simulink library "AEMS_Standard_Library"  (R2016b)
settings: Solver=ode45  StartTime=0.0  StopTime=10.0  RelTol=1e-3
undefined symbols (not defined in the file or in its folder): BkPY, carto, Cbx_extegr, Cbx_lpegrsys, Cbx_portegr, Cnx_bnk_nr_conf, Cnx_cyl_nr_conf, ConfigManagement, configuration_management, Cxx_dcm_io_tmr_end_xxxx, Cxx_dcm_rt_tmr_end, Cxx_DID_xxxx_IO_max, Cxx_DID_xxxx_IO_min, Cxx_egrhsofs, Cxx_vmaniegi, DEM_DEBOUNCE_FREEZE, DEM_DTR_CTL_INVISIBLE, DEM_DTR_CTL_NORMAL, Dem_DtrId2_XXX, Dem_DtrId3_XXX, Dem_DtrId4_XXX, Dem_DtrId5_XXX, Dem_DtrId6_XXX, Dem_DtrId7_XXX, Dem_DtrId8_XXX, Dem_DtrId9_XXX, Dem_DtrId_XXX, Dem_EnableConditionId2_XXX, Dem_EnableConditionId3_XXX, Dem_EnableConditionId4_XXX, Dem_EnableConditionId5_XXX, Dem_EnableConditionId6_XXX, Dem_EnableConditionId7_XXX, Dem_EnableConditionId8_XXX, Dem_EnableConditionId_XXX, Dem_EventId, Dem_EventId2_XXX, Dem_EventId3_XXX, Dem_EventId4_XXX, Dem_EventId5_XXX, Dem_EventId6_XXX, Dem_EventId7_XXX, Dem_EventId8_XXX, Dem_EventId9_XXX, Dem_EventId_Device_Faulttype, Dem_EventId_XXX, DEM_IUMPR_GENERAL_DENOMINATOR, DEM_OPCYC_IGNITION, Dem_RatioId2_XXX, Dem_RatioId3_XXX, Dem_RatioId4_XXX, Dem_RatioId5_XXX, Dem_RatioId6_XXX, Dem_RatioId7_XXX, Dem_RatioId8_XXX, Dem_RatioId_XXX, Dem_StorageConditionId2_XXX, Dem_StorageConditionId3_XXX, Dem_StorageConditionId4_XXX, Dem_StorageConditionId5_XXX ... (+65)
libraries: AEMS_Standard_Library x477, simulink x2
(part 38 of 39)

== system AEMS_Standard_Library/SPECIFIC/AEMS_AT_EHR/A_Enabled_Calculation/B_Temp_calculation_in_brick/C_Temp_and_power_calculation ==
  Vxx_ehr_exo_temp_flu : Inport
  Vxx_ehr_wht_temp_flu : Inport  Port=2
  Vxx_ehr_ex_gas_temp_flu : Inport  Port=3
  Vxx_ehr_ext_cnvt_temp_flu : Inport  Port=4
  Vxx_ehr_sel_tenv : Inport  Port=5
  Vxx_ehr_samp_t : Inport  Port=6
  Vxx_ehr_ext_cnvt_entr : Inport  Port=7
  Constant1 : Constant  Value=0  OutDataTypeStr=Inherit: Inherit via back propagation
  DivisionByZero : Subsystem
  Product2 : Product  OutDataTypeStr=Inherit: Inherit via back propagation  RndMeth=Zero
  Saturation : Saturate  UpperLimit=1473  LowerLimit=233  RndMeth=Zero
      settings: AttributesFormatString=<limits=%<UpperLimit>/%<LowerLimit>>
  Sum : Sum  Inputs=+-  OutDataTypeStr=Inherit: Inherit via back propagation  RndMeth=Zero  InputSameDT=on
  Sum1 : Sum  Inputs=2  OutDataTypeStr=Inherit: Inherit via back propagation  RndMeth=Zero  InputSameDT=on
  Sum2 : Sum  Inputs=2  OutDataTypeStr=Inherit: Inherit via back propagation  RndMeth=Zero  InputSameDT=on
  Sum3 : Sum  Inputs=2  OutDataTypeStr=Inherit: Inherit via back propagation  RndMeth=Zero  InputSameDT=on
  Vxx_ehr_ext_pow_loss : Outport
  Vxx_ehr_dtp : Outport  Port=2
  wires:
  Saturation/1 -> Vxx_ehr_dtp/1, Sum/1
  Sum3/1 -> Saturation/1
  Sum2/1 -> Sum3/2
  Sum1/1 -> Sum3/1
  Vxx_ehr_ext_cnvt_entr/1 -> DivisionByZero/2(Vxx_ehr_ext_cnvt_entr)
  Vxx_ehr_samp_t/1 -> DivisionByZero/1(Vxx_ehr_samp_t)
  Vxx_ehr_sel_tenv/1 -> Sum/2
  Sum/1 -> Product2/1
  DivisionByZero/1(ans) -> Product2/2
  Product2/1 -> Vxx_ehr_ext_pow_loss/1
  Vxx_ehr_exo_temp_flu/1 -> Sum1/1
  Vxx_ehr_wht_temp_flu/1 -> Sum1/2
  Vxx_ehr_ex_gas_temp_flu/1 -> Sum2/1
  Vxx_ehr_ext_cnvt_temp_flu/1 -> Sum2/2
  Constant1/1 -> DivisionByZero/3(ans_of_0div)

== system AEMS_Standard_Library/SPECIFIC/AEMS_AT_TUBE/A_Thermal_Calculation/B_Thermal_Material_Model_Tube/DivisionByZero ==
  Vxx_tub_samp_t : Inport
  num : Inport  Port=2
  ans_of_0div : Inport  Port=3
  Divide : Product  Inputs=*/  OutDataTypeStr=Inherit: Inherit via back propagation  RndMeth=Zero
  MinMax1 : MinMax  Function=max  Inputs=2  OutDataTypeStr=Inherit: Inherit via back propagation  RndMeth=Zero  InputSameDT=on
  RelationalOperator : RelationalOperator  Operator=~=  OutDataTypeStr=boolean  RndMeth=Nearest  InputSameDT=on
  Switch1 : Switch  Criteria=u2 ~= 0  RndMeth=Zero  SaturateOnIntegerOverflow=on  InputSameDT=on
      settings: AttributesFormatString=Criteria=%<Criteria>
  imm_zero : Constant  Value=0  OutDataTypeStr=Inherit: Inherit via back propagation
  imm_zero3 : Constant  Value=Den_Tol  OutDataTypeStr=Inherit: Inherit via back propagation
  Vxx_tub_temp_pow_loss : Outport
  wires:
  RelationalOperator/1 -> Switch1/2
  imm_zero/1 -> RelationalOperator/2
  Switch1/1 -> Vxx_tub_temp_pow_loss/1
  num/1 -> Divide/1
  Divide/1 -> Switch1/1
  ans_of_0div/1 -> Switch1/3
  Vxx_tub_samp_t/1 -> RelationalOperator/1, MinMax1/1
  MinMax1/1 -> Divide/2
  imm_zero3/1 -> MinMax1/2

== system AEMS_Standard_Library/SPECIFIC/AEMS_AT_TUBE/A_Thermal_Calculation/B_Thermal_Material_Model_Tube/DivisionByZero1 ==
  Vxx_tub_entr_tot : Inport
  Vxx_tub_ext_cnvt_entr : Inport  Port=2
  ans_of_0div : Inport  Port=3
  Divide : Product  Inputs=*/  OutDataTypeStr=Inherit: Inherit via back propagation  RndMeth=Zero
  MinMax1 : MinMax  Function=max  Inputs=2  OutDataTypeStr=Inherit: Inherit via back propagation  RndMeth=Zero  InputSameDT=on
  RelationalOperator : RelationalOperator  Operator=~=  OutDataTypeStr=boolean  RndMeth=Nearest  InputSameDT=on
  Switch1 : Switch  Criteria=u2 ~= 0  RndMeth=Zero  SaturateOnIntegerOverflow=on  InputSameDT=on
      settings: AttributesFormatString=Criteria=%<Criteria>
  imm_zero : Constant  Value=0  OutDataTypeStr=Inherit: Inherit via back propagation
  imm_zero3 : Constant  Value=Den_Tol  OutDataTypeStr=Inherit: Inherit via back propagation
  ans : Outport
  wires:
  imm_zero3/1 -> MinMax1/2
  MinMax1/1 -> Divide/2
  Vxx_tub_entr_tot/1 -> MinMax1/1, RelationalOperator/1
  ans_of_0div/1 -> Switch1/3
  Divide/1 -> Switch1/1
  Vxx_tub_ext_cnvt_entr/1 -> Divide/1
  Switch1/1 -> ans/1
  imm_zero/1 -> RelationalOperator/2
  RelationalOperator/1 -> Switch1/2

== system AEMS_Standard_Library/SPECIFIC/AEMS_AT_TUBE/A_Thermal_Calculation/B_Thermal_Material_Model_Tube/DivisionByZero2 ==
  Vxx_tub_entr_tot : Inport
  Vxx_tub_itl_cnvt_entr : Inport  Port=2
  ans_of_0div : Inport  Port=3
  Divide : Product  Inputs=*/  OutDataTypeStr=Inherit: Inherit via back propagation  RndMeth=Zero
  MinMax1 : MinMax  Function=max  Inputs=2  OutDataTypeStr=Inherit: Inherit via back propagation  RndMeth=Zero  InputSameDT=on
  RelationalOperator : RelationalOperator  Operator=~=  OutDataTypeStr=boolean  RndMeth=Nearest  InputSameDT=on
  Switch1 : Switch  Criteria=u2 ~= 0  RndMeth=Zero  SaturateOnIntegerOverflow=on  InputSameDT=on
      settings: AttributesFormatString=Criteria=%<Criteria>
  imm_zero : Constant  Value=0  OutDataTypeStr=Inherit: Inherit via back propagation
  imm_zero3 : Constant  Value=Den_Tol  OutDataTypeStr=Inherit: Inherit via back propagation
  ans : Outport
  wires:
  RelationalOperator/1 -> Switch1/2
  imm_zero/1 -> RelationalOperator/2
  Switch1/1 -> ans/1
  Vxx_tub_itl_cnvt_entr/1 -> Divide/1
  Divide/1 -> Switch1/1
  ans_of_0div/1 -> Switch1/3
  Vxx_tub_entr_tot/1 -> RelationalOperator/1, MinMax1/1
  MinMax1/1 -> Divide/2
  imm_zero3/1 -> MinMax1/2

== system AEMS_Standard_Library/SPECIFIC/AEMS_AT_TUBE/A_Thermal_Calculation/B_Thermal_Material_Model_Tube/DivisionByZero3 ==
  Vxx_tub_entr_tot : Inport
  Vxx_tub_wht_entr : Inport  Port=2
  ans_of_0div : Inport  Port=3
  Divide : Product  Inputs=*/  OutDataTypeStr=Inherit: Inherit via back propagation  RndMeth=Zero
  MinMax1 : MinMax  Function=max  Inputs=2  OutDataTypeStr=Inherit: Inherit via back propagation  RndMeth=Zero  InputSameDT=on
  RelationalOperator : RelationalOperator  Operator=~=  OutDataTypeStr=boolean  RndMeth=Nearest  InputSameDT=on
  Switch1 : Switch  Criteria=u2 ~= 0  RndMeth=Zero  SaturateOnIntegerOverflow=on  InputSameDT=on
      settings: AttributesFormatString=Criteria=%<Criteria>
  imm_zero : Constant  Value=0  OutDataTypeStr=Inherit: Inherit via back propagation
  imm_zero3 : Constant  Value=Den_Tol  OutDataTypeStr=Inherit: Inherit via back propagation
  ans : Outport
  wires:
  imm_zero3/1 -> MinMax1/2
  MinMax1/1 -> Divide/2
  Vxx_tub_entr_tot/1 -> MinMax1/1, RelationalOperator/1
  ans_of_0div/1 -> Switch1/3
  Divide/1 -> Switch1/1
  Vxx_tub_wht_entr/1 -> Divide/1
  Switch1/1 -> ans/1
  imm_zero/1 -> RelationalOperator/2
  RelationalOperator/1 -> Switch1/2

== system AEMS_Standard_Library/SPECIFIC/AEMS_AT_TUBE/A_Thermal_Calculation/C_Thermal_Gas_Model_Tube/DivisionByZero1 ==
  Vxx_tub_gas_entr_tot : Inport
  Vxx_tub_ex_gas_entr : Inport  Port=2
  ans_of_0div : Inport  Port=3
  Divide : Product  Inputs=*/  OutDataTypeStr=Inherit: Inherit via back propagation  RndMeth=Zero
  MinMax1 : MinMax  Function=max  Inputs=2  OutDataTypeStr=Inherit: Inherit via back propagation  RndMeth=Zero  InputSameDT=on
  RelationalOperator : RelationalOperator  Operator=~=  OutDataTypeStr=boolean  RndMeth=Nearest  InputSameDT=on
  Switch1 : Switch  Criteria=u2 ~= 0  RndMeth=Zero  SaturateOnIntegerOverflow=on  InputSameDT=on
      settings: AttributesFormatString=Criteria=%<Criteria>
  imm_zero : Constant  Value=0  OutDataTypeStr=Inherit: Inherit via back propagation
  imm_zero3 : Constant  Value=Den_Tol  OutDataTypeStr=Inherit: Inherit via back propagation
  ans : Outport
  wires:
  imm_zero3/1 -> MinMax1/2
  MinMax1/1 -> Divide/2
  Vxx_tub_gas_entr_tot/1 -> MinMax1/1, RelationalOperator/1
  ans_of_0div/1 -> Switch1/3
  Divide/1 -> Switch1/1
  Vxx_tub_ex_gas_entr/1 -> Divide/1
  Switch1/1 -> ans/1
  imm_zero/1 -> RelationalOperator/2
  RelationalOperator/1 -> Switch1/2

== system AEMS_Standard_Library/SPECIFIC/AEMS_AT_TUBE/A_Thermal_Calculation/C_Thermal_Gas_Model_Tube/DivisionByZero2 ==
  Vxx_tub_samp_t : Inport
  num : Inport  Port=2
  ans_of_0div : Inport  Port=3
  Divide : Product  Inputs=*/  OutDataTypeStr=Inherit: Inherit via back propagation  RndMeth=Zero
  MinMax1 : MinMax  Function=max  Inputs=2  OutDataTypeStr=Inherit: Inherit via back propagation  RndMeth=Zero  InputSameDT=on
  RelationalOperator : RelationalOperator  Operator=~=  OutDataTypeStr=boolean  RndMeth=Nearest  InputSameDT=on
  Switch1 : Switch  Criteria=u2 ~= 0  RndMeth=Zero  SaturateOnIntegerOverflow=on  InputSameDT=on
      settings: AttributesFormatString=Criteria=%<Criteria>
  imm_zero : Constant  Value=0  OutDataTypeStr=Inherit: Inherit via back propagation
  imm_zero3 : Constant  Value=Den_Tol  OutDataTypeStr=Inherit: Inherit via back propagation
  Vxx_tub_ex_gas_pow_loss : Outport
  wires:
  imm_zero3/1 -> MinMax1/2
  MinMax1/1 -> Divide/2
  Vxx_tub_samp_t/1 -> MinMax1/1, RelationalOperator/1
  ans_of_0div/1 -> Switch1/3
  Divide/1 -> Switch1/1
  num/1 -> Divide/1
  Switch1/1 -> Vxx_tub_ex_gas_pow_loss/1
  imm_zero/1 -> RelationalOperator/2
  RelationalOperator/1 -> Switch1/2

== system AEMS_Standard_Library/SPECIFIC/AEMS_AT_TUBE/A_Thermal_Calculation/C_Thermal_Gas_Model_Tube/DivisionByZero3 ==
  Vxx_tub_gas_entr_tot : Inport
  Vxx_tub_itl_gas_wht_entr : Inport  Port=2
  ans_of_0div : Inport  Port=3
  Divide : Product  Inputs=*/  OutDataTypeStr=Inherit: Inherit via back propagation  RndMeth=Zero
  MinMax1 : MinMax  Function=max  Inputs=2  OutDataTypeStr=Inherit: Inherit via back propagation  RndMeth=Zero  InputSameDT=on
  RelationalOperator : RelationalOperator  Operator=~=  OutDataTypeStr=boolean  RndMeth=Nearest  InputSameDT=on
  Switch1 : Switch  Criteria=u2 ~= 0  RndMeth=Zero  SaturateOnIntegerOverflow=on  InputSameDT=on
      settings: AttributesFormatString=Criteria=%<Criteria>
  imm_zero : Constant  Value=0  OutDataTypeStr=Inherit: Inherit via back propagation
  imm_zero3 : Constant  Value=Den_Tol  OutDataTypeStr=Inherit: Inherit via back propagation
  ans : Outport
  wires:
  RelationalOperator/1 -> Switch1/2
  imm_zero/1 -> RelationalOperator/2
  Switch1/1 -> ans/1
  Vxx_tub_itl_gas_wht_entr/1 -> Divide/1
  Divide/1 -> Switch1/1
  ans_of_0div/1 -> Switch1/3
  Vxx_tub_gas_entr_tot/1 -> RelationalOperator/1, MinMax1/1
  MinMax1/1 -> Divide/2
  imm_zero3/1 -> MinMax1/2

== system AEMS_Standard_Library/SPECIFIC/AEMS_AT_TUBE/A_Thermal_Calculation/C_Thermal_Gas_Model_Tube/DivisionByZero4 ==
  Vxx_tub_gas_entr_tot : Inport
  num : Inport  Port=2
  ans_of_0div : Inport  Port=3
  Divide : Product  Inputs=*/  OutDataTypeStr=Inherit: Inherit via back propagation  RndMeth=Zero
  MinMax1 : MinMax  Function=max  Inputs=2  OutDataTypeStr=Inherit: Inherit via back propagation  RndMeth=Zero  InputSameDT=on
  RelationalOperator : RelationalOperator  Operator=~=  OutDataTypeStr=boolean  RndMeth=Nearest  InputSameDT=on
  Switch1 : Switch  Criteria=u2 ~= 0  RndMeth=Zero  SaturateOnIntegerOverflow=on  InputSameDT=on
      settings: AttributesFormatString=Criteria=%<Criteria>
  imm_zero : Constant  Value=0  OutDataTypeStr=Inherit: Inherit via back propagation
  imm_zero3 : Constant  Value=Den_Tol  OutDataTypeStr=Inherit: Inherit via back propagation
  Vxx_tub_gas_itl_cnvt_entr_rat : Outport
  wires:
  imm_zero3/1 -> MinMax1/2
  MinMax1/1 -> Divide/2
  Vxx_tub_gas_entr_tot/1 -> MinMax1/1, RelationalOperator/1
  ans_of_0div/1 -> Switch1/3
  Divide/1 -> Switch1/1
  num/1 -> Divide/1
  Switch1/1 -> Vxx_tub_gas_itl_cnvt_entr_rat/1
  imm_zero/1 -> RelationalOperator/2
  RelationalOperator/1 -> Switch1/2

== system AEMS_Standard_Library/SPECIFIC/AEMS_AT_TUBE/A_Thermal_Calculation/C_Thermal_Gas_Model_Tube/DivisionByZero5 ==
  Vxx_tub_gas_entr_tot : Inport
  num : Inport  Port=2
  ans_of_0div : Inport  Port=3
  Divide : Product  Inputs=*/  OutDataTypeStr=Inherit: Inherit via back propagation  RndMeth=Zero
  MinMax1 : MinMax  Function=max  Inputs=2  OutDataTypeStr=Inherit: Inherit via back propagation  RndMeth=Zero  InputSameDT=on
  RelationalOperator : RelationalOperator  Operator=~=  OutDataTypeStr=boolean  RndMeth=Nearest  InputSameDT=on
  Switch1 : Switch  Criteria=u2 ~= 0  RndMeth=Zero  SaturateOnIntegerOverflow=on  InputSameDT=on
      settings: AttributesFormatString=Criteria=%<Criteria>
  imm_zero : Constant  Value=0  OutDataTypeStr=Inherit: Inherit via back propagation
  imm_zero3 : Constant  Value=Den_Tol  OutDataTypeStr=Inherit: Inherit via back propagation
  Vxx_tub_gas_utp_wht_entr_rat : Outport
  wires:
  RelationalOperator/1 -> Switch1/2
  imm_zero/1 -> RelationalOperator/2
  Switch1/1 -> Vxx_tub_gas_utp_wht_entr_rat/1
  num/1 -> Divide/1
  Divide/1 -> Switch1/1
  ans_of_0div/1 -> Switch1/3
  Vxx_tub_gas_entr_tot/1 -> RelationalOperator/1, MinMax1/1
  MinMax1/1 -> Divide/2
  imm_zero3/1 -> MinMax1/2

== system AEMS_Standard_Library/SPECIFIC/AEMS_AT_TUBE/A_Thermal_Calculation/C_Thermal_Gas_Model_Tube/DivisionByZero6 ==
  Vxx_tub_gas_entr_tot : Inport
  num : Inport  Port=2
  ans_of_0div : Inport  Port=3
  Divide : Product  Inputs=*/  OutDataTypeStr=Inherit: Inherit via back propagation  RndMeth=Zero
  MinMax1 : MinMax  Function=max  Inputs=2  OutDataTypeStr=Inherit: Inherit via back propagation  RndMeth=Zero  InputSameDT=on
  RelationalOperator : RelationalOperator  Operator=~=  OutDataTypeStr=boolean  RndMeth=Nearest  InputSameDT=on
  Switch1 : Switch  Criteria=u2 ~= 0  RndMeth=Zero  SaturateOnIntegerOverflow=on  InputSameDT=on
      settings: AttributesFormatString=Criteria=%<Criteria>
  imm_zero : Constant  Value=0  OutDataTypeStr=Inherit: Inherit via back propagation
  imm_zero3 : Constant  Value=Den_Tol  OutDataTypeStr=Inherit: Inherit via back propagation
  ans : Outport
  wires:
  imm_zero3/1 -> MinMax1/2
  MinMax1/1 -> Divide/2
  Vxx_tub_gas_entr_tot/1 -> MinMax1/1, RelationalOperator/1
  ans_of_0div/1 -> Switch1/3
  Divide/1 -> Switch1/1
  num/1 -> Divide/1
  Switch1/1 -> ans/1
  imm_zero/1 -> RelationalOperator/2
  RelationalOperator/1 -> Switch1/2

== system AEMS_Standard_Library/SPECIFIC/AEMS_AS_PADE/A_pade_model/A_filter_pade/A_filter_1/A_pade_2nd_order_filter_1 ==
  Vxx_b0_1 : Inport
  Vxx_b1_1 : Inport  Port=2
  Vxx_b2_1 : Inport  Port=3
  Vxx_a1_1 : Inport  Port=4
  Vxx_a2_1 : Inport  Port=5
  Vxx_in_fil : Inport  Port=6
  Vbx_dly_init_ena : Inport  Port=7
  AEMS_UNITDELAY_RESET_EXTERNALIC{,1..3} (4 alike) : AEMS_Standard_Library/DISCRETE/AEMS_UNITDELAY_RESET_EXTERNALIC  Tag=[LIB]
      settings: AttributesFormatString=%<MaskType>
  Product{,1..2,4..5} (5 alike) : Product  OutDataTypeStr=Inherit: Inherit via back propagation  RndMeth=Zero
  Saturation{,1,3..4} (4 alike) : Saturate  UpperLimit=1  LowerLimit=-2  RndMeth=Zero
      settings: AttributesFormatString=<limits=%<UpperLimit>/%<LowerLimit>>
  Saturation2 : Saturate  UpperLimit=1.5  LowerLimit=0  RndMeth=Zero
      settings: AttributesFormatString=<limits=%<UpperLimit>/%<LowerLimit>>
  Sum : Sum  OutDataTypeStr=Inherit: Inherit via back propagation  RndMeth=Zero  InputSameDT=on
  Sum1 : Sum  OutDataTypeStr=Inherit: Inherit via back propagation  RndMeth=Zero  InputSameDT=on
  Sum2 : Sum  Inputs=|+-  OutDataTypeStr=Inherit: Inherit via back propagation  RndMeth=Zero  InputSameDT=on
  Sum3 : Sum  OutDataTypeStr=Inherit: Inherit via back propagation  RndMeth=Zero  InputSameDT=on
  Vxx_dly_1 : Outport
  wires:
  Product5/1 -> Sum1/1
  AEMS_UNITDELAY_RESET_EXTERNALIC2/1 -> Product5/2
  Sum/1 -> Sum3/1
  AEMS_UNITDELAY_RESET_EXTERNALIC3/1 -> Product4/2, AEMS_UNITDELAY_RESET_EXTERNALIC2/1
  Product2/1 -> Sum3/2
  AEMS_UNITDELAY_RESET_EXTERNALIC1/1 -> Product2/1
  Product1/1 -> Sum/2
  AEMS_UNITDELAY_RESET_EXTERNALIC/1 -> Product1/1, AEMS_UNITDELAY_RESET_EXTERNALIC1/1
  Vbx_dly_init_ena/1 -> AEMS_UNITDELAY_RESET_EXTERNALIC2/2, AEMS_UNITDELAY_RESET_EXTERNALIC3/2, AEMS_UNITDELAY_RESET_EXTERNALIC1/2, AEMS_UNITDELAY_RESET_EXTERNALIC/2
  Sum1/1 -> Sum2/2
  Vxx_in_fil/1 -> Product/1, AEMS_UNITDELAY_RESET_EXTERNALIC2/3, AEMS_UNITDELAY_RESET_EXTERNALIC3/3, AEMS_UNITDELAY_RESET_EXTERNALIC1/3, AEMS_UNITDELAY_RESET_EXTERNALIC/3, AEMS_UNITDELAY_RESET_EXTERNALIC/1
  Vxx_b0_1/1 -> Saturation/1
  Vxx_b1_1/1 -> Saturation1/1
  Vxx_b2_1/1 -> Saturation2/1
  Product/1 -> Sum/1
  Sum2/1 -> AEMS_UNITDELAY_RESET_EXTERNALIC3/1, Vxx_dly_1/1
  Vxx_a2_1/1 -> Saturation3/1
  Product4/1 -> Sum1/2
  Vxx_a1_1/1 -> Saturation4/1
  Saturation/1 -> Product/2
  Saturation1/1 -> Product1/2
  Saturation2/1 -> Product2/2
  Saturation3/1 -> Product5/1
  Saturation4/1 -> Product4/1
  Sum3/1 -> Sum2/1

== system AEMS_Standard_Library/SPECIFIC/AEMS_AS_PADE/A_pade_model/A_filter_pade/B_filter_2/A_pade_2nd_order_filter_2 ==
  Vxx_b0_2 : Inport
  Vxx_b1_2 : Inport  Port=2
  Vxx_b2_2 : Inport  Port=3
  Vxx_a1_2 : Inport  Port=4
  Vxx_a2_2 : Inport  Port=5
  Vxx_dly_1 : Inport  Port=6
  Vbx_dly_init_ena : Inport  Port=7
  Vxx_in_fil : Inport  Port=8
  AEMS_UNITDELAY_RESET_EXTERNALIC{,1..3} (4 alike) : AEMS_Standard_Library/DISCRETE/AEMS_UNITDELAY_RESET_EXTERNALIC  Tag=[LIB]
      settings: AttributesFormatString=%<MaskType>
  Product{,1..2,4..5} (5 alike) : Product  OutDataTypeStr=Inherit: Inherit via back propagation  RndMeth=Zero
  Saturation{,1,3..4} (4 alike) : Saturate  UpperLimit=1  LowerLimit=-2  RndMeth=Zero
      settings: AttributesFormatString=<limits=%<UpperLimit>/%<LowerLimit>>
  Saturation2 : Saturate  UpperLimit=1.5  LowerLimit=0  RndMeth=Zero
      settings: AttributesFormatString=<limits=%<UpperLimit>/%<LowerLimit>>
  Sum : Sum  OutDataTypeStr=Inherit: Inherit via back propagation  RndMeth=Zero  InputSameDT=on
  Sum1 : Sum  Inputs=|++  OutDataTypeStr=Inherit: Inherit via back propagation  RndMeth=Zero  InputSameDT=on
  Sum2 : Sum  Inputs=|+-  OutDataTypeStr=Inherit: Inherit via back propagation  RndMeth=Zero  InputSameDT=on
  Sum3 : Sum  OutDataTypeStr=Inherit: Inherit via back propagation  RndMeth=Zero  InputSameDT=on
  Vxx_dly_2 : Outport
  wires:
  Vxx_in_fil/1 -> AEMS_UNITDELAY_RESET_EXTERNALIC2/3, AEMS_UNITDELAY_RESET_EXTERNALIC3/3, AEMS_UNITDELAY_RESET_EXTERNALIC1/3, AEMS_UNITDELAY_RESET_EXTERNALIC/3
  Product4/1 -> Sum1/2
  Product5/1 -> Sum1/1
  AEMS_UNITDELAY_RESET_EXTERNALIC2/1 -> Product5/1
  Sum/1 -> Sum3/1
  AEMS_UNITDELAY_RESET_EXTERNALIC3/1 -> Product4/1, AEMS_UNITDELAY_RESET_EXTERNALIC2/1
  AEMS_UNITDELAY_RESET_EXTERNALIC1/1 -> Product2/1
  Product1/1 -> Sum/2
  AEMS_UNITDELAY_RESET_EXTERNALIC/1 -> Product1/1, AEMS_UNITDELAY_RESET_EXTERNALIC1/1
  Vbx_dly_init_ena/1 -> AEMS_UNITDELAY_RESET_EXTERNALIC/2, AEMS_UNITDELAY_RESET_EXTERNALIC1/2, AEMS_UNITDELAY_RESET_EXTERNALIC2/2, AEMS_UNITDELAY_RESET_EXTERNALIC3/2
  Sum1/1 -> Sum2/2
  Vxx_dly_1/1 -> Product/1, AEMS_UNITDELAY_RESET_EXTERNALIC/1
  Vxx_b0_2/1 -> Saturation/1
  Vxx_b2_2/1 -> Saturation2/1
  Product/1 -> Sum/1
  Sum2/1 -> Vxx_dly_2/1, AEMS_UNITDELAY_RESET_EXTERNALIC3/1
  Vxx_a1_2/1 -> Saturation4/1
  Vxx_b1_2/1 -> Saturation1/1
  Vxx_a2_2/1 -> Saturation3/1
  Saturation/1 -> Product/2
  Saturation1/1 -> Product1/2
  Saturation2/1 -> Product2/2
  Saturation3/1 -> Product5/2
  Saturation4/1 -> Product4/2
  Product2/1 -> Sum3/2
  Sum3/1 -> Sum2/1

== system AEMS_Standard_Library/SPECIFIC/AEMS_AS_PADE/A_pade_model/A_filter_pade/C_filter_3/A_pade_2nd_order_filter_3 ==
  Vxx_b0_3 : Inport
  Vxx_b1_3 : Inport  Port=2
  Vxx_b2_3 : Inport  Port=3
  Vxx_a1_3 : Inport  Port=4
  Vxx_a2_3 : Inport  Port=5
  Vxx_dly_2 : Inport  Port=6
  Vbx_dly_init_ena : Inport  Port=7
  Vxx_in_fil : Inport  Port=8
  AEMS_UNITDELAY_RESET_EXTERNALIC{,1..3} (4 alike) : AEMS_Standard_Library/DISCRETE/AEMS_UNITDELAY_RESET_EXTERNALIC  Tag=[LIB]
      settings: AttributesFormatString=%<MaskType>
  Product{,1..2,4..5} (5 alike) : Product  OutDataTypeStr=Inherit: Inherit via back propagation  RndMeth=Zero
  Saturation{,1,3..4} (4 alike) : Saturate  UpperLimit=1  LowerLimit=-2  RndMeth=Zero
      settings: AttributesFormatString=<limits=%<UpperLimit>/%<LowerLimit>>
  Saturation2 : Saturate  UpperLimit=1.5  LowerLimit=0  RndMeth=Zero
      settings: AttributesFormatString=<limits=%<UpperLimit>/%<LowerLimit>>
  Sum : Sum  OutDataTypeStr=Inherit: Inherit via back propagation  RndMeth=Zero  InputSameDT=on
  Sum1 : Sum  Inputs=|++  OutDataTypeStr=Inherit: Inherit via back propagation  RndMeth=Zero  InputSameDT=on
  Sum2 : Sum  Inputs=|+-  OutDataTypeStr=Inherit: Inherit via back propagation  RndMeth=Zero  InputSameDT=on
  Sum3 : Sum  OutDataTypeStr=Inherit: Inherit via back propagation  RndMeth=Zero  InputSameDT=on
  Vxx_in_dly : Outport
  wires:
  Vxx_in_fil/1 -> AEMS_UNITDELAY_RESET_EXTERNALIC/3, AEMS_UNITDELAY_RESET_EXTERNALIC2/3, AEMS_UNITDELAY_RESET_EXTERNALIC3/3, AEMS_UNITDELAY_RESET_EXTERNALIC1/3
  Product4/1 -> Sum1/2
  Product5/1 -> Sum1/1
  AEMS_UNITDELAY_RESET_EXTERNALIC2/1 -> Product5/2
  Sum/1 -> Sum3/1
  AEMS_UNITDELAY_RESET_EXTERNALIC3/1 -> AEMS_UNITDELAY_RESET_EXTERNALIC2/1, Product4/1
  Product2/1 -> Sum3/2
  AEMS_UNITDELAY_RESET_EXTERNALIC1/1 -> Product2/1
  Product1/1 -> Sum/2
  AEMS_UNITDELAY_RESET_EXTERNALIC/1 -> Product1/1, AEMS_UNITDELAY_RESET_EXTERNALIC1/1
  Vbx_dly_init_ena/1 -> AEMS_UNITDELAY_RESET_EXTERNALIC2/2, AEMS_UNITDELAY_RESET_EXTERNALIC3/2, AEMS_UNITDELAY_RESET_EXTERNALIC1/2, AEMS_UNITDELAY_RESET_EXTERNALIC/2
  Sum1/1 -> Sum2/2
  Vxx_dly_2/1 -> Product/1, AEMS_UNITDELAY_RESET_EXTERNALIC/1
  Vxx_b0_3/1 -> Saturation/1
  Vxx_b1_3/1 -> Saturation1/1
  Vxx_b2_3/1 -> Saturation2/1
  Product/1 -> Sum/1
  Sum2/1 -> Vxx_in_dly/1, AEMS_UNITDELAY_RESET_EXTERNALIC3/1
  Vxx_a1_3/1 -> Saturation4/1
  Vxx_a2_3/1 -> Saturation3/1
  Saturation/1 -> Product/2
  Saturation1/1 -> Product1/2
  Saturation2/1 -> Product2/2
  Saturation3/1 -> Product5/1
  Saturation4/1 -> Product4/2
  Sum3/1 -> Sum2/1

== system AEMS_Standard_Library/SPECIFIC/AEMS_AT_EHR/A_Enabled_Calculation/B_Temp_calculation_in_brick/A_Entropy_calculation/DivisionByZero ==
  Vxx_ehr_entr_tot : Inport
  num : Inport  Port=2
  ans_of_0div : Inport  Port=3
  Divide : Product  Inputs=*/  OutDataTypeStr=Inherit: Inherit via back propagation  RndMeth=Zero
  MinMax1 : MinMax  Function=max  Inputs=2  OutDataTypeStr=Inherit: Inherit via back propagation  RndMeth=Zero  InputSameDT=on
  RelationalOperator : RelationalOperator  Operator=~=  OutDataTypeStr=boolean  RndMeth=Nearest  InputSameDT=on
  Switch1 : Switch  Criteria=u2 ~= 0  RndMeth=Zero  SaturateOnIntegerOverflow=on  InputSameDT=on
      settings: AttributesFormatString=Criteria=%<Criteria>
  imm_zero : Constant  Value=0  OutDataTypeStr=Inherit: Inherit via back propagation
  imm_zero3 : Constant  Value=Den_Tol  OutDataTypeStr=Inherit: Inherit via back propagation
  Vxx_ehr_wht_entr_rat : Outport
  wires:
  RelationalOperator/1 -> Switch1/2
  imm_zero/1 -> RelationalOperator/2
  Switch1/1 -> Vxx_ehr_wht_entr_rat/1
  num/1 -> Divide/1
  Divide/1 -> Switch1/1
  ans_of_0div/1 -> Switch1/3
  Vxx_ehr_entr_tot/1 -> MinMax1/1, RelationalOperator/1
  MinMax1/1 -> Divide/2
  imm_zero3/1 -> MinMax1/2

== system AEMS_Standard_Library/SPECIFIC/AEMS_AT_EHR/A_Enabled_Calculation/B_Temp_calculation_in_brick/A_Entropy_calculation/DivisionByZero1 ==
  Vxx_ehr_entr_tot : Inport
  num : Inport  Port=2
  ans_of_0div : Inport  Port=3
  Divide : Product  Inputs=*/  OutDataTypeStr=Inherit: Inherit via back propagation  RndMeth=Zero
  MinMax1 : MinMax  Function=max  Inputs=2  OutDataTypeStr=Inherit: Inherit via back propagation  RndMeth=Zero  InputSameDT=on
  RelationalOperator : RelationalOperator  Operator=~=  OutDataTypeStr=boolean  RndMeth=Nearest  InputSameDT=on
  Switch1 : Switch  Criteria=u2 ~= 0  RndMeth=Zero  SaturateOnIntegerOverflow=on  InputSameDT=on
      settings: AttributesFormatString=Criteria=%<Criteria>
  imm_zero : Constant  Value=0  OutDataTypeStr=Inherit: Inherit via back propagation
  imm_zero3 : Constant  Value=Den_Tol  OutDataTypeStr=Inherit: Inherit via back propagation
  Vxx_ehr_ex_gas_entr_rat : Outport
  wires:
  imm_zero3/1 -> MinMax1/2
  MinMax1/1 -> Divide/2
  Vxx_ehr_entr_tot/1 -> RelationalOperator/1, MinMax1/1
  ans_of_0div/1 -> Switch1/3
  Divide/1 -> Switch1/1
  num/1 -> Divide/1
  Switch1/1 -> Vxx_ehr_ex_gas_entr_rat/1
  imm_zero/1 -> RelationalOperator/2
  RelationalOperator/1 -> Switch1/2

== system AEMS_Standard_Library/SPECIFIC/AEMS_AT_EHR/A_Enabled_Calculation/B_Temp_calculation_in_brick/A_Entropy_calculation/DivisionByZero2 ==
  Vxx_ehr_entr_tot : Inport
  num : Inport  Port=2
  ans_of_0div : Inport  Port=3
  Divide : Product  Inputs=*/  OutDataTypeStr=Inherit: Inherit via back propagation  RndMeth=Zero
  MinMax1 : MinMax  Function=max  Inputs=2  OutDataTypeStr=Inherit: Inherit via back propagation  RndMeth=Zero  InputSameDT=on
  RelationalOperator : RelationalOperator  Operator=~=  OutDataTypeStr=boolean  RndMeth=Nearest  InputSameDT=on
  Switch1 : Switch  Criteria=u2 ~= 0  RndMeth=Zero  SaturateOnIntegerOverflow=on  InputSameDT=on
      settings: AttributesFormatString=Criteria=%<Criteria>
  imm_zero : Constant  Value=0  OutDataTypeStr=Inherit: Inherit via back propagation
  imm_zero3 : Constant  Value=Den_Tol  OutDataTypeStr=Inherit: Inherit via back propagation
  Vxx_ehr_ext_cnvt_entr_rat : Outport
  wires:
  RelationalOperator/1 -> Switch1/2
  imm_zero/1 -> RelationalOperator/2
  Switch1/1 -> Vxx_ehr_ext_cnvt_entr_rat/1
  num/1 -> Divide/1
  Divide/1 -> Switch1/1
  ans_of_0div/1 -> Switch1/3
  Vxx_ehr_entr_tot/1 -> MinMax1/1, RelationalOperator/1
  MinMax1/1 -> Divide/2
  imm_zero3/1 -> MinMax1/2

== system AEMS_Standard_Library/SPECIFIC/AEMS_AT_EHR/A_Enabled_Calculation/B_Temp_calculation_in_brick/B_Temp_fluctuation_calculation/DivisionByZero ==
  Vxx_ehr_entr_tot : Inport
  num : Inport  Port=2
  ans_of_0div : Inport  Port=3
  Divide : Product  Inputs=*/  OutDataTypeStr=Inherit: Inherit via back propagation  RndMeth=Zero
  MinMax1 : MinMax  Function=max  Inputs=2  OutDataTypeStr=Inherit: Inherit via back propagation  RndMeth=Zero  InputSameDT=on
  RelationalOperator : RelationalOperator  Operator=~=  OutDataTypeStr=boolean  RndMeth=Nearest  InputSameDT=on
  Switch1 : Switch  Criteria=u2 ~= 0  RndMeth=Zero  SaturateOnIntegerOverflow=on  InputSameDT=on
      settings: AttributesFormatString=Criteria=%<Criteria>
  imm_zero : Constant  Value=0  OutDataTypeStr=Inherit: Inherit via back propagation
  imm_zero3 : Constant  Value=Den_Tol  OutDataTypeStr=Inherit: Inherit via back propagation
  Vxx_ehr_exo_temp_flu : Outport
  wires:
  imm_zero3/1 -> MinMax1/2
  MinMax1/1 -> Divide/2
  Vxx_ehr_entr_tot/1 -> RelationalOperator/1, MinMax1/1
  ans_of_0div/1 -> Switch1/3
  Divide/1 -> Switch1/1
  num/1 -> Divide/1
  Switch1/1 -> Vxx_ehr_exo_temp_flu/1
  imm_zero/1 -> RelationalOperator/2
  RelationalOperator/1 -> Switch1/2

== system AEMS_Standard_Library/SPECIFIC/AEMS_AT_EHR/A_Enabled_Calculation/B_Temp_calculation_in_brick/C_Temp_and_power_calculation/DivisionByZero ==
  Vxx_ehr_samp_t : Inport
  Vxx_ehr_ext_cnvt_entr : Inport  Port=2
  ans_of_0div : Inport  Port=3
  Divide : Product  Inputs=*/  OutDataTypeStr=Inherit: Inherit via back propagation  RndMeth=Zero
  MinMax1 : MinMax  Function=max  Inputs=2  OutDataTypeStr=Inherit: Inherit via back propagation  RndMeth=Zero  InputSameDT=on
  RelationalOperator : RelationalOperator  Operator=~=  OutDataTypeStr=boolean  RndMeth=Nearest  InputSameDT=on
  Switch1 : Switch  Criteria=u2 ~= 0  RndMeth=Zero  SaturateOnIntegerOverflow=on  InputSameDT=on
      settings: AttributesFormatString=Criteria=%<Criteria>
  imm_zero : Constant  Value=0  OutDataTypeStr=Inherit: Inherit via back propagation
  imm_zero3 : Constant  Value=Den_Tol  OutDataTypeStr=Inherit: Inherit via back propagation
  ans : Outport
  wires:
  imm_zero3/1 -> MinMax1/2
  MinMax1/1 -> Divide/2
  Vxx_ehr_samp_t/1 -> RelationalOperator/1, MinMax1/1
  ans_of_0div/1 -> Switch1/3
  Divide/1 -> Switch1/1
  Vxx_ehr_ext_cnvt_entr/1 -> Divide/1
  Switch1/1 -> ans/1
  imm_zero/1 -> RelationalOperator/2
  RelationalOperator/1 -> Switch1/2

== stateflow chart AEMS_Standard_Library/BIT_OPERATION/AEMS_BITWISEAND/Chart ==
  (default) -> (junction 2) : {Out=(uint32(Input_data)&uint32(Mask));}
  data: Input_data input; Mask input; Out output type(Input_data)

== stateflow chart AEMS_Standard_Library/BIT_OPERATION/AEMS_BITWISEOR/Chart ==
  (default) -> (junction 2) : {Out=(uint32(Input_data)|uint32(Mask));}
  data: Input_data input; Mask input; Out output type(Input_data)

== stateflow chart AEMS_Standard_Library/BIT_OPERATION/AEMS_BITWISEXOR/Chart ==
  (default) -> (junction 2) : {Out=(uint32(Input_data)^uint32(Mask));}
  data: Input_data input; Mask input; Out output type(Input_data)

== stateflow chart AEMS_Standard_Library/BIT_OPERATION/AEMS_BIT_GET/Chart ==
  (default) -> (junction 2) : {x=1c;
      | Bit_value=(uint32(In)&(x<<uint8(Bit_number)))!=0;}
  data: In input; Bit_number input; Bit_value output boolean; x local uint32

== stateflow chart AEMS_Standard_Library/BIT_OPERATION/AEMS_EXTRACT_BIT/Chart ==
  (default) -> (junction 2) : {Bit_value=( (In & Bit_number) / RH);}
  data: In input; Bit_number input; Bit_value output u_inp_data; RH input

== stateflow chart AEMS_Standard_Library/BIT_OPERATION/AEMS_BIT_SET16/Chart ==
  (default) -> (junction 17) : {Out =uint8(Bit1)+ uint8(Bit2)* 2+uint8(Bit3)* 4+uint8(Bit4)* 8+uint8(Bit5)* 16+uint8(Bit6)* 32+uint8(Bit7)* 64+uint8(Bit8)* 128 + uint8(Bit9)* 256+ uint8(Bit10)* 512+uint8(Bit11)* 1024+uint8(Bit12)* 2048+uint8(Bit13)* 4096+uint8(Bit14)* 8192+uint8(Bit15)* 16384+uint8(Bit16)* 32768;}
  data: Bit1 input; Bit2 input; Bit3 input; Bit4 input; Bit5 input; Bit6 input; Bit7 input; Bit8 input; Out output uint16; Bit9 input; Bit10 input; Bit11 input; Bit12 input; Bit13 input; Bit14 input; Bit15 input; Bit16 input

== stateflow chart AEMS_Standard_Library/BIT_OPERATION/AEMS_BIT_SET8/Chart ==
  (default) -> (junction 17) : {Out =uint8(Bit1)+ uint8(Bit2)* 2+uint8(Bit3)* 4+uint8(Bit4)* 8+uint8(Bit5)* 16+uint8(Bit6)* 32+uint8(Bit7)* 64+uint8(Bit8)* 128;}
  data: Bit1 input; Bit2 input; Bit3 input; Bit4 input; Bit5 input; Bit6 input; Bit7 input; Bit8 input; Out output uint8

== stateflow chart AEMS_Standard_Library/BIT_OPERATION/AEMS_CONVERT_TO_UNSIGNED_SI/Chart ==
  (default) -> (junction 2) : {Bit_value=(In & Mask);}
  data: In input; Bit_value output; Mask input

== stateflow chart AEMS_Standard_Library/SUB/AEMS_CONVERT_BUFFER_TO_FLP/Chart1 ==
  note: Is_Negative : Based on the The MSB of the Input_Buffer, Negativity is prdicted for signed integers
      | NOTE: Input_Buff is in the order MSB first.i.e. 6500 -> 0xFDE8. Input_Buff[0] => 0xFD; Input_Buff[1]=>0xE8
  note: //If the ctrl reaches here means
      | DataType is 6//(uint32)
  note: Perform 1's complement ; Performing ExOR operation with any number & 255 will give teh 1s complement of that number.
  note: Perform 2's complement
  (default) -> (junction 2) : {
      | Mask_Buff[0] = 1;
      | Mask_Buff[1] = 256;
      | Mask_Buff[2] = 65536;
      | Mask_Buff[3] = 16777216 ;
      | Idx = 0;
      | Fxp_Scalar_Value  = 0.0;
      | IsProgress_2sComplement_Conv = 1;
      | }
  (junction 2) -> (junction 4) [order 1] : [DataType == 1]   //If data type is int8
  (junction 2) -> (junction 38) [order 2]
  (junction 4) -> (junction 33) : {
      | Num_Byte = 1;
      | Is_Negative= Input_Buff[0] & 128;
      | }
  (junction 38) -> (junction 46) [order 1] : [DataType == 2]   //If data type is uint8
  (junction 38) -> (junction 81) [order 2]
  (junction 46) -> (junction 45) : {
      | Num_Byte = 1;
      | Is_Negative=0;
      | }
  (junction 81) -> (junction 82) [order 1] : [DataType ==3] //If data type is int16
  (junction 81) -> (junction 85) [order 2]
  (junction 82) -> (junction 83) : {
      | Num_Byte = 2;
      | Is_Negative= Input_Buff[0] & 128;
      | }
  (junction 85) -> (junction 86) [order 1] : [DataType ==4] //If data type is uint16
  (junction 85) -> (junction 89) [order 2]
  (junction 86) -> (junction 87) : {
      | Num_Byte = 2;
      | Is_Negative=0;
      | }
  (junction 89) -> (junction 90) [order 1] : [DataType ==5] //If data type is int32
  (junction 89) -> (junction 93) [order 2] : {
      | Num_Byte = 4;
      | Is_Negative=0;
      | }
  (junction 90) -> (junction 91) : {
      | Num_Byte = 4;
      | Is_Negative= Input_Buff[0] & 128;
      | }
  (junction 91) -> (junction 93)
  (junction 87) -> (junction 91)
  (junction 83) -> (junction 87)
  (junction 45) -> (junction 83)
  (junction 33) -> (junction 45)
  (junction 93) -> (junction 215)
  (junction 215) -> (junction 217) [order 1] : [Idx < Num_Byte]
  (junction 219) -> (junction 215) : {Idx = Idx +1;}
  (junction 215) -> (junction 107) [order 2] : {Idx = 0;}
  (junction 217) -> (junction 219) : {Temp_Input_Buff[Idx] =Input_Buff[Idx];}
  (junction 107) -> (junction 110) [order 1] : [Is_Negative ~= 0]
  (junction 107) -> (junction 180) [order 2]
  (junction 110) -> (junction 113)
  (junction 113) -> (junction 116) [order 1] : [Idx<Num_Byte]
  (junction 198) -> (junction 113) : {Idx = Idx +1;}
  (junction 113) -> (junction 153) [order 2] : {Idx = Num_Byte - 1;}
  (junction 116) -> (junction 198) : {Temp_Input_Buff[Idx] = Temp_Input_Buff[Idx] ^ 255;}
  (junction 153) -> (junction 157) [order 1] : [Idx >= 0]
  (junction 176) -> (junction 153) : {Idx = Idx - 1;}
  (junction 153) -> (junction 181) [order 2]
  (junction 157) -> (junction 162)
  (junction 162) -> (junction 163) [order 1] : [Temp_Input_Buff [Idx] == 255 && IsProgress_2sComplement_Conv]
  (junction 162) -> (junction 168) [order 2]
  (junction 163) -> (junction 166) : {
      | Temp_Input_Buff [Idx]=0;
      | }
  (junction 168) -> (junction 172) [order 1] : [IsProgress_2sComplement_Conv]
  (junction 168) -> (junction 176) [order 2]
  (junction 172) -> (junction 173) : {
      | Temp_Input_Buff [Idx]= Temp_Input_Buff [Idx] + 1;
      | IsProgress_2sComplement_Conv=0;
      | }
  (junction 173) -> (junction 176)
  (junction 166) -> (junction 173)
  (junction 181) -> (junction 180)
  (junction 180) -> (junction 190) : {
      | Idx = 0;
      | }
  (junction 190) -> (junction 191) [order 1] : [Idx<Num_Byte]
  (junction 192) -> (junction 190) : {Idx = Idx +1;}
  (junction 190) -> (junction 134) [order 2]
  (junction 191) -> (junction 192) : {
      | Fxp_Scalar_Value = Fxp_Scalar_Value + single((Temp_Input_Buff[Num_Byte-Idx-1] * Mask_Buff[Idx] ));
      | }
  (junction 134) -> (junction 137) [order 1] : [Is_Negative ~= 0]
  (junction 134) -> (junction 140) [order 2]
  (junction 137) -> (junction 138) : {Fxp_Scalar_Value = (-1.0 * Fxp_Scalar_Value);}
  (junction 138) -> (junction 140)
  (junction 140) -> (junction 144)
  data: DataType input uint8; Mask_Buff local uint32 size=4 =[0 0 0 0]; Num_Byte local uint8; Is_Negative local uint32; Idx local int8; Input_Buff input uint8; Temp_Input_Buff local uint8 size=4 =[0 0 0 0]; IsProgress_2sComplement_Conv local boolean; Fxp_Scalar_Value output single

== stateflow chart AEMS_Standard_Library/SUB/AEMS_CONVERT_BYTE_TO_FLP/Chart1 ==
  note: Is_Negative : Based on the The MSB of the Input_Buffer, Negativity is prdicted for signed integers
      | NOTE: Input_Buff is in the order MSB first.i.e. 6500 -> 0xFDE8. Input_Buff[0] => 0xFD; Input_Buff[1]=>0xE8
  note: If the ctrl reaches here
      | means it's uint8
  note: Performs Bitwise Not (Any number ^(ExOR) with 255 gives 1s complement
  note: Perform 2's complement
  (default) -> (junction 2) : {
      | Fxp_Scalar_Value  = 0.0;
      | Temp_Input = Input;
      | }
  (junction 2) -> (junction 4) [order 1] : [DataType == 1]   //If data type is int8
  (junction 2) -> (junction 81) [order 2] : {
      | Is_Negative=0;
      | }
  (junction 4) -> (junction 33) : {
      | Is_Negative= Input & 128;
      | }
  (junction 33) -> (junction 81)
  (junction 81) -> (junction 107)
  (junction 107) -> (junction 110) [order 1] : [Is_Negative ~= 0]
  (junction 110) -> (junction 225) : { Temp_Input = Temp_Input ^ 255;}
  (junction 107) -> (junction 180) [order 2] : {Fxp_Scalar_Value = single(Temp_Input);}
  (junction 225) -> (junction 227) [order 1] : [Temp_Input == 255]
  (junction 225) -> (junction 231) [order 2] : {
      | Temp_Input = Temp_Input + 1;
      | Fxp_Scalar_Value = single(-1*Temp_Input);
      | }
  (junction 227) -> (junction 229) : {Fxp_Scalar_Value= 0.0;}
  (junction 229) -> (junction 231)
  (junction 231) -> (junction 180)
  (junction 180) -> (junction 236)
  data: DataType input uint8; Is_Negative local uint32; Input input uint8; Temp_Input local uint8 =0; Fxp_Scalar_Value output single

== stateflow chart AEMS_Standard_Library/SPECIFIC/AEMS_LOOKUP_LIBRARY/Lookup_library ==
  (default) -> (junction 147)
  (junction 147) -> (junction 110) : {
      | index=0;
      | ratio=0;
      | }
  (junction 110) -> (junction 104) [order 1] : [brk_pt[len_tbl-1] <= ref_val  ]
  (junction 104) -> (junction 123) : {
      | dlt1 = 1;
      | dlt2 = 1;
      | output_hi =  tbl[len_tbl-1];
      | output_lo =  tbl[len_tbl-1];
      | }
  (junction 110) -> (junction 132) [order 2]
  (junction 132) -> (junction 134)
  (junction 134) -> (junction 116) [order 1] : [brk_pt[0] >= ref_val  ]
  (junction 116) -> (junction 124) : {
      | dlt1 = 1;
      | dlt2 = 1;
      | output_hi =  tbl[0];
      | output_lo =  tbl[0];
      | }
  (junction 134) -> (junction 136) [order 2]
  (junction 136) -> (junction 10)
  (junction 10) -> (junction 100) [order 1] : [(index < len_tbl) &&...
      |  (brk_pt[index] < ref_val) ]
  (junction 100) -> (junction 112) : {index++;}
  (junction 112) -> (junction 10)
  (junction 10) -> (junction 101) [order 2]
  (junction 101) -> (junction 106) : {
      | dlt1 = (ref_val - brk_pt[index-1]);
      | dlt2 = (brk_pt[index] - brk_pt[index-1]);
      | output_hi =  tbl[index];
      | output_lo =  tbl[index-1];
      | }
  (junction 106) -> (junction 131)
  (junction 123) -> (junction 124)
  (junction 124) -> (junction 131)
  (junction 131) -> (junction 121)
  data: ref_val input single size=1; tbl input single; brk_pt input single; output_hi output single size=1 =0; index local uint8 size=1 =0; ratio local single size=1 =0; len_tbl input uint8 size=1; dlt1 output single size=1 =1; dlt2 output single size=1 =1; output_lo output single size=1 =0

== stateflow chart AEMS_Standard_Library/SPECIFIC/AEMS_OL_RATE_COUNTER/OL_RATE_COUNTER ==
  (default) -> (junction 25)
  (junction 25) -> (junction 42)
  (junction 42) -> (junction 43) [order 1] : [ fdata_clear ]
  (junction 42) -> (junction 26) [order 2]
  (junction 43) -> (junction 41) : {
      | vrate_denominator = 0;
      | vrate_numerator = 0;
      | }
  (junction 26) -> (junction 27) [order 1] : [ frate_denominator && ~festrp ]
  (junction 26) -> (junction 29) [order 2]
  (junction 27) -> (junction 28) : {
      | vrate_denominator ++;
      | festrp = 1;
      | }
  (junction 28) -> (junction 29)
  (junction 29) -> (junction 34)
  (junction 34) -> (junction 31)
  (junction 31) -> (junction 32) [order 1] : [ frate_numerator && ~fcntend ]
  (junction 31) -> (junction 30) [order 2]
  (junction 32) -> (junction 33) : {
      | vrate_numerator ++;
      | fcntend = 1;
      | }
  (junction 33) -> (junction 30)
  (junction 30) -> (junction 35)
  (junction 35) -> (junction 36)
  (junction 36) -> (junction 37) [order 1] : [ (vrate_denominator > 65534) || (vrate_numerator > 65534) ]
  (junction 36) -> (junction 39) [order 2]
  (junction 37) -> (junction 38) : {
      | vrate_denominator /= 2.0;
      | vrate_numerator /= 2.0;
      | }
  (junction 38) -> (junction 39)
  (junction 39) -> (junction 44)
  (junction 41) -> (junction 44)
  (junction 44) -> (junction 40)
  data: frate_numerator input boolean size=1; fcntend output boolean size=1 =0; festrp output boolean size=1 =0; frate_denominator input boolean size=1; fdata_clear input boolean size=1; vrate_numerator output uint16 size=1 =0; vrate_denominator output uint16 size=1 =0

== stateflow chart AEMS_Standard_Library/SPECIFIC/AEMS_DGN_MF_MISX_CALCULATION_LIB/DGN_MF_misx_calcuration_lib_AEMS ==
  (default) -> (junction 23)
  (junction 23) -> (junction 24) : {
      | vtint_pre_diff = vtint_num_mem[index_base] - vtint_num_mem[index_pre] ;
      | vmisx_num_pre = vtint_pre_times * vtint_pre_diff ;
      |
      | vtint_post_diff = vtint_num_mem[index_base] - vtint_num_mem[index_post] ;
      | vmisx_num_post = vtint_post_times * vtint_post_diff ;
      |
      | vmisx_num = vmisx_num_pre + vmisx_num_post ;
      | }
  (junction 24) -> (junction 21) : {
      | vtint_den_sqr = vtint_den_mem[index_den] * vtint_den_mem[index_den] ;
      | vtint_den_cube = vtint_den_mem[index_den] * vtint_den_sqr ;
      |
      | vtp_msec = vtp * 1000 ;
      | vmisx_den_tmp = vtint_den_cube * vtp_msec ;
      | vmisx_den = vmisx_den_tmp * vmisxhos ;
      | }
  (junction 21) -> (junction 25) [order 1] : [ (vmisx_den >= 0.001) ]
  (junction 21) -> (junction 22) [order 2]
  (junction 25) -> (junction 31) : {
      | vmisx_org = vmisx_num / vmisx_den;
      | vmisx_tmp = vmisx_org * mmsu ;
      | }
  (junction 31) -> (junction 32) [order 1] : [ vmisx_tmp < -128 ]
  (junction 31) -> (junction 34) [order 2]
  (junction 32) -> (junction 33) : {
      | vmisx = -128 ;
      | }
  (junction 22) -> (junction 27) [order 1] : [ (vmisx_num >= 0) ]
  (junction 34) -> (junction 35) [order 1] : [ vmisx_tmp <= 127 ]
  (junction 22) -> (junction 29) [order 2] : {
      | vmisx = -128 ;
      | }
  (junction 27) -> (junction 28) : {
      | vmisx = 127 ;
      | }
  (junction 34) -> (junction 26) [order 2] : {
      | vmisx = 127 ;
      | }
  (junction 35) -> (junction 36) : {
      | vmisx = vmisx_tmp ;
      | }
  (junction 28) -> (junction 29)
  (junction 36) -> (junction 26)
  (junction 33) -> (junction 36)
  (junction 26) -> (junction 28)
  (junction 29) -> (junction 30)
  data: vtint_den_mem input single size=18; vtint_num_mem input single size=18; index_base input uint8 size=1; index_pre input uint8 size=1; index_post input uint8 size=1; index_den input uint8 size=1; vtint_pre_times input uint8 size=1 =0; vtint_post_times input uint8 size=1 =0; mmsu input single size=1; vtp input single size=1; vmisx output single size=1 =0; vmisx_den local single size=1 =0; vmisx_den_tmp local single size=1 =0; vmisx_num local single size=1 =0; vmisx_num_post local single size=1 =0; vmisx_num_pre local single size=1 =0; vmisx_org local single size=1 =0; vmisxhos input single size=1; vtint_den_cube local single size=1 =0; vtint_den_sqr local single size=1 =0; vtint_post_diff local single size=1 =0; vtint_pre_diff local single size=1 =0; vtp_msec local single size=1 =0; vmisx_tmp local single size=1 =0

== stateflow chart AEMS_Standard_Library/SPECIFIC/AEMS_OL_SIMILAR_CONDITION_SET/OL_SIMILAR_CONDITION_SET ==
  (default) -> (junction 20)
  (junction 20) -> (junction 51)
  (junction 51) -> (junction 53) [order 1] : [ initialize == 0 ]
  (junction 53) -> (junction 55) : {
      | pending_hold = pending ;
      | mil_hold = mil ;
      | initialize = 1 ;
      | }
  (junction 51) -> (junction 57) [order 2]
  (junction 55) -> (junction 57)
  (junction 57) -> (junction 60)
  (junction 60) -> (junction 21)
  (junction 21) -> (junction 25) [order 1] : [ mil == 1 ]
  (junction 21) -> (junction 22) [order 2]
  (junction 25) -> (junction 62)
  (junction 22) -> (junction 23) [order 1] : [ erase == 1 ]
  (junction 22) -> (junction 80) [order 2]
  (junction 23) -> (junction 77) : {
      | similar_engine_rev = 0 ;
      | similar_load_value = 0 ;
      | similar_coolant_temp = -50 ;
      | mil_hold = 0 ;
      | rewrite_hold = 0 ;
      | pending_hold = 0 ;
      | }
  (junction 80) -> (junction 82) [order 1] : [  rewrite == 1 ]
  (junction 80) -> (junction 29) [order 2]
  (junction 82) -> (junction 84)
  (junction 29) -> (junction 30) [order 1] : [ pending == 1 ]
  (junction 29) -> (junction 27) [order 2]
  (junction 30) -> (junction 70)
  (junction 62) -> (junction 65) [order 1] : [ mil_hold == 0 ]
  (junction 70) -> (junction 72) [order 1] : [ pending_hold == 0 ]
  (junction 84) -> (junction 86) [order 1] : [ rewrite_hold == 0  ]
  (junction 65) -> (junction 67) : {
      | similar_engine_rev = engine_rev ;
      | similar_load_value = load_value ;
      | similar_coolant_temp = coolant_temp ;
      | mil_hold = 1 ;
      | }
  (junction 70) -> (junction 31) [order 2]
  (junction 72) -> (junction 74) : {
      | similar_engine_rev = engine_rev ;
      | similar_load_value = load_value ;
      | similar_coolant_temp = coolant_temp ;
      | pending_hold = 1 ;
      | }
  (junction 84) -> (junction 91) [order 2]
  (junction 86) -> (junction 88) : {
      | similar_engine_rev = engine_rev ;
      | similar_load_value = load_value ;
      | similar_coolant_temp = coolant_temp ;
      | rewrite_hold = 1 ;
      | }
  (junction 62) -> (junction 26) [order 2]
  (junction 31) -> (junction 27)
  (junction 74) -> (junction 31)
  (junction 91) -> (junction 74)
  (junction 88) -> (junction 91)
  (junction 77) -> (junction 88)
  (junction 26) -> (junction 77)
  (junction 67) -> (junction 26)
  (junction 27) -> (junction 28) : {
      | similar_condition_set = (pending_hold || mil_hold) ;
      | }
  data: similar_condition_set output boolean size=1 =0; mil_hold local boolean size=1 =0; similar_engine_rev output size=1 =0; similar_load_value output size=1 =0; erase input boolean size=1; mil input boolean size=1; pending input boolean size=1; rewrite input boolean size=1; engine_rev input size=1; load_value input size=1; coolant_temp input size=1; similar_coolant_temp output size=1 =-50; rewrite_hold local boolean size=1 =0; initialize local boolean size=1 =0; pending_hold local boolean size=1 =0

== stateflow chart AEMS_Standard_Library/SPECIFIC/AEMS_EGRQESTH_SELECT_AND_TRIM_LIB/M2002_2A_2A_0x_EGR_DELAY_NR_10ms ==
  (default) -> (junction 39)
  (junction 39) -> (junction 36)
  (junction 36) -> (junction 35) : {
      | delaytimer=egrtgstdly+0.000001
      | }
  (junction 40) -> (junction 42) [order 1] : [46>count]
  (junction 42) -> (junction 46) : {
      | temptime=count*0.01;
      | counta=count+1;
      | temptimea=counta*0.01;
      | }
  (junction 35) -> (junction 33) [order 1] : [delaytimer>=0.005]
  (junction 33) -> (junction 30) [order 1] : [delaytimer<0.45]
  (junction 35) -> (junction 38) [order 2] : {
      | delaycount=0;
      | }
  (junction 33) -> (junction 37) [order 2] : {
      | delaycount=45;
      | }
  (junction 30) -> (junction 49)
  (junction 49) -> (junction 40) : {
      | count=1;
      | }
  (junction 46) -> (junction 44) [order 1] : [(temptime-0.005 <= delaytimer)&&(delaytimer < temptimea-0.005)]
  (junction 46) -> (junction 45) [order 2]
  (junction 44) -> (junction 43) : {
      | delaycount=count;
      | }
  (junction 47) -> (junction 40) : {
      | count++;
      | }
  (junction 40) -> (junction 48) [order 2]
  (junction 43) -> (junction 45)
  (junction 45) -> (junction 47)
  (junction 48) -> (junction 51)
  (junction 51) -> (junction 50)
  (junction 37) -> (junction 38)
  (junction 50) -> (junction 37)
  (junction 38) -> (junction 53)
  (junction 53) -> (junction 34) : {
      | num=45;
      | }
  (junction 34) -> (junction 32) [order 1] : [0<num]
  (junction 32) -> (junction 31) : {
      | temp[num]=temp[num-1];
      | }
  (junction 31) -> (junction 34) : {
      | num--;
      | }
  (junction 34) -> (junction 41) [order 2] : {
      | temp[0]=vegrqcohx_nr0;
      | egrqcohbl=temp[delaycount];
      | }
  (junction 41) -> (junction 52)
  data: vegrqcohx_nr0 input; egrtgstdly input; egrqcohbl output single =0; delaycount local uint8 =0; num local uint8 =0; temp local single size=46 =0; count local uint8 =0; delaytimer local single =0; counta local uint8 =0; temptime local single =0; temptimea local single =0

== stateflow chart AEMS_Standard_Library/SPECIFIC/AEMS_OL_RATE_COUNTER_B/OL_RATE_COUNTER_B ==
  (default) -> (junction 33)
  (junction 33) -> (junction 57)
  (junction 57) -> (junction 56) [order 1] : [ fdata_clear ]
  (junction 57) -> (junction 41) [order 2]
  (junction 56) -> (junction 55) : {
      | vrate_denominator = 0;
      | vrate_numerator = 0;
      | }
  (junction 54) -> (junction 49) [order 1] : [ index <= 2 ]
  (junction 41) -> (junction 54) : {
      | index = 1;
      | }
  (junction 49) -> (junction 42)
  (junction 42) -> (junction 34)
  (junction 34) -> (junction 35) [order 1] : [ frate_denominator[index] && ~festrp[index] ]
  (junction 34) -> (junction 37) [order 2]
  (junction 35) -> (junction 36) : {
      | vrate_denominator[index] ++;
      | festrp[index] = 1;
      | }
  (junction 36) -> (junction 37)
  (junction 37) -> (junction 58)
  (junction 58) -> (junction 39)
  (junction 39) -> (junction 40) [order 1] : [ frate_numerator[index] && ~fcntend[index] ]
  (junction 39) -> (junction 38) [order 2]
  (junction 40) -> (junction 50) : {
      | vrate_numerator[index] ++;
      | fcntend[index] = 1;
      | }
  (junction 51) -> (junction 54) : {
      | index ++;
      | }
  (junction 54) -> (junction 43) [order 2]
  (junction 50) -> (junction 38)
  (junction 38) -> (junction 48)
  (junction 48) -> (junction 44)
  (junction 44) -> (junction 45) [order 1] : [ (vrate_denominator[index] > 65534) || (vrate_numerator[index] > 65534) ]
  (junction 44) -> (junction 47) [order 2]
  (junction 45) -> (junction 46) : {
      | vrate_denominator[index] /= 2.0;
      | vrate_numerator[index] /= 2.0;
      | }
  (junction 46) -> (junction 47)
  (junction 47) -> (junction 59)
  (junction 59) -> (junction 51)
  (junction 43) -> (junction 53)
  (junction 55) -> (junction 53)
  (junction 53) -> (junction 52)
  data: frate_numerator input boolean size=2; fcntend output boolean size=2 =0; festrp output boolean size=2 =0; frate_denominator input boolean size=2; fdata_clear input boolean size=1; vrate_numerator output uint16 size=2 =0; vrate_denominator output uint16 size=2 =0; index local uint8 size=1 =1
